simulink subsystem "rp_dac"  (R2021a)
settings: Solver=VariableStepAuto  StartTime=0.0  StopTime=10.0  RelTol=1e-3
libraries: xbsIndex_r4 x6, xps_library x3
settings Model: Creator=casper  LastModifiedBy=casper

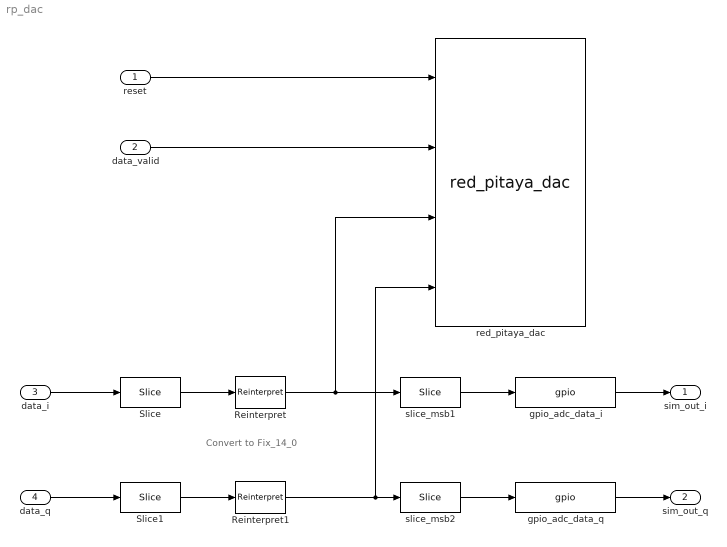
== system rp_dac ==
  note: Convert to Fix_14_0
  reset : Inport
  data_valid : Inport  Port=2
  data_i : Inport  Port=3
  data_q : Inport  Port=4
  Reinterpret : xbsIndex_r4/Reinterpret  force_arith_type=on  arith_type="Signed  (2's comp)"  force_bin_pt=off  bin_pt=0  block_type=reinterpret
  Reinterpret1 : xbsIndex_r4/Reinterpret  force_arith_type=on  arith_type="Signed  (2's comp)"  force_bin_pt=off  bin_pt=0  block_type=reinterpret
  Slice : xbsIndex_r4/Slice  nbits=14  boolean_output=off  mode=Upper Bit Location + Width  bit1=0  base1=MSB of Input  bit0=0  base0=LSB of Input  dbl_ovrd=off  block_type=slice
  Slice1 : xbsIndex_r4/Slice  nbits=14  boolean_output=off  mode=Upper Bit Location + Width  bit1=0  base1=MSB of Input  bit0=0  base0=LSB of Input  dbl_ovrd=off  block_type=slice
  gpio_adc_data_i : xps_library/IO/gpio  Tag=xps:gpio  io_group_params_forwarded=on  io_group=ROACH2:led  io_group_real=gpio  io_group_custom=0  io_dir=out  arith_type="Signed  (2's comp)"  bitwidth=8  bin_pt=0  bit_index=[0,1,2,3,4,5,6,7]  sample_period=1  use_single_ended=off  use_ddr=off  reg_iob=on  reg_clk_phase=0  termination=None  use_iodelay=off
      settings: SourceProductName=CASPER XPS Blockset
  gpio_adc_data_q : xps_library/IO/gpio  Tag=xps:gpio  io_group_params_forwarded=on  io_group=ROACH2:led  io_group_real=gpio  io_group_custom=0  io_dir=out  arith_type="Signed  (2's comp)"  bitwidth=8  bin_pt=0  bit_index=[8,9,10,11,12,13,14,15]  sample_period=1  use_single_ended=off  use_ddr=off  reg_iob=on  reg_clk_phase=0  termination=None  use_iodelay=off
      settings: SourceProductName=CASPER XPS Blockset
  red_pitaya_dac : xps_library/DACs/red_pitaya_dac  Tag=xps:red_pitaya_dac  bits=14
      settings: SourceProductName=CASPER XPS Blockset
  slice_msb1 : xbsIndex_r4/Slice  nbits=8  boolean_output=off  mode=Upper Bit Location + Width  bit1=0  base1=MSB of Input  bit0=0  base0=LSB of Input  dbl_ovrd=off  block_type=slice
  slice_msb2 : xbsIndex_r4/Slice  nbits=8  boolean_output=off  mode=Upper Bit Location + Width  bit1=0  base1=MSB of Input  bit0=0  base0=LSB of Input  dbl_ovrd=off  block_type=slice
  sim_out_i : Outport
  sim_out_q : Outport  Port=2
  wires:
  gpio_adc_data_q/1 -> sim_out_q/1
  data_q/1 -> Slice1/1
  slice_msb2/1 -> gpio_adc_data_q/1
  data_valid/1 -> red_pitaya_dac/2
  gpio_adc_data_i/1 -> sim_out_i/1
  Reinterpret1/1 -> red_pitaya_dac/4, slice_msb2/1
  slice_msb1/1 -> gpio_adc_data_i/1
  data_i/1 -> Slice/1
  reset/1 -> red_pitaya_dac/1
  Slice/1 -> Reinterpret/1
  Reinterpret/1 -> red_pitaya_dac/3, slice_msb1/1
  Slice1/1 -> Reinterpret1/1
